simulink model "CruiseControl"  (R2020b)
settings: Solver=ode45  StartTime=0.0  StopTime=10  RelTol=1e-3
values from neighbouring files (symbols this model uses):
  b = 50.0    [Dictionary.sldd]
  m = 1000.0    [Dictionary.sldd]
settings Model: DataDictionary=Dictionary.sldd  OrderedModelArguments=off  Creator=abhin  LastModifiedBy=abhin

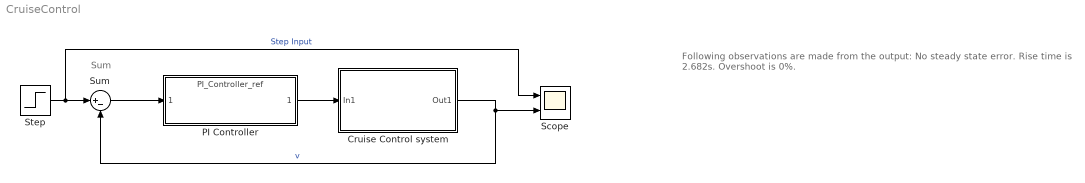
== system CruiseControl ==
  note: Following observations are made from the output:
      | No steady state error.
      | Rise time is 2.682s.
      | Overshoot is 0%.
  note: Sum
  Cruise Control system : Subsystem
  PI Controller : ModelReference  ModelNameDialog=PI_Controller_ref  SimulationMode=Normal  ModelReferenceVersion=1.7
  Scope : Scope  NumInputPorts=2
  Step : Step  After=500  SampleTime=0
  Sum : Sum  Inputs=|+-
  wires:
  Step/1 -> Scope/1, Sum/1  "Step Input"
  Cruise Control system/1(Out1) -> Scope/2, Sum/2  "v"
  PI Controller/1 -> Cruise Control system/1(In1)
  Sum/1 -> PI Controller/1

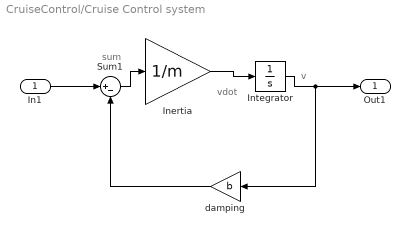
== system CruiseControl/Cruise Control system ==
  note: v
  note: sum
  note: vdot
  In1 : Inport  OutDataTypeStr=double  PortDimensions=1  SampleTime=0
  Inertia : Gain  Gain=1/m
  Integrator : Integrator
  Sum1 : Sum  Inputs=|+-
  damping : Gain  Gain=b
  Out1 : Outport  OutDataTypeStr=double  PortDimensions=1  SampleTime=0
  wires:
  Inertia/1 -> Integrator/1
  Sum1/1 -> Inertia/1
  Integrator/1 -> Out1/1, damping/1
  In1/1 -> Sum1/1
  damping/1 -> Sum1/2
